simulink model "amplSim_2012b"  (R2012b)
settings: Solver=ode15s  StartTime=0.0  StopTime=30  RelTol=1e-6
values from neighbouring files (symbols this model uses):
  K = par(4)    [amplDiff.m]
  Qin = C*U    (= 2.912e-09)    [amplDiff.m]
  t0 = par(1)    [amplDiff.m]
  tau1 = par(2)    [amplDiff.m]
  tau2 = par(3)    [amplDiff.m]
  y_off = par(5)    [amplDiff.m]    (also in approxVol.m = theta(5))
settings Model: Creator=larer  LastModifiedBy=larer
settings DataIOCC: SignalLoggingSaveFormat=ModelDataLogs  SignalLoggingName=sigsOut
settings OptimizationCC: BooleanDataType=off  ExpressionDepthLimit=128
settings DebuggingCC: SaveWithParameterizedLinksMsg=none  SignalResolutionControl=TryResolveAllWithWarning  SolverPrmCheckMsg=none  MultiTaskDSMMsg=warning  MultiTaskCondExecSysMsg=none  FrameProcessingCompatibilityMsg=error  StateNameClashWarn=none  StrictBusMsg=None
settings HardwareCC: TargetUnknown=on
settings CodeAppCC: CustomSymbolStrType=$N$R$M_T
settings GRTTargetCC: CodeReplacementLibrary=C89/C90 (ANSI)  GeneratePreprocessorConditionals=Use local settings  CombineOutputUpdateFcns=off  GRTInterface=on

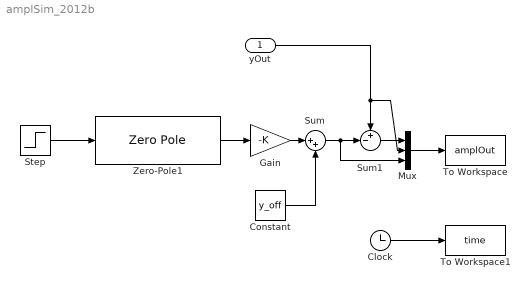
== system amplSim_2012b ==
  yOut : Inport
  Clock : Clock
  Constant : Constant  Value=y_off
  Gain : Gain  Gain=-K  SaturateOnIntegerOverflow=on  OutDataTypeStr=Inherit: Same as input  ParamDataTypeStr=Inherit: Same as input
  Mux : Mux  Inputs=3
  Step : Step  Time=t0  After=Qin  SampleTime=0
  Sum : Sum  Inputs=|++  SaturateOnIntegerOverflow=on  InputSameDT=on  OutDataTypeStr=Inherit: Same as first input
  Sum1 : Sum  Inputs=+-|  SaturateOnIntegerOverflow=on  InputSameDT=on  OutDataTypeStr=Inherit: Same as first input
  To Workspace : ToWorkspace  VariableName=amplOut  SampleTime=0.01
  To Workspace1 : ToWorkspace  VariableName=time  SampleTime=0.01
  Zero-Pole1 : ZeroPole  Zeros=[0]  Poles=[-1/tau1 -1/tau2]  Gain=[1/tau2/tau1]
  wires:
  Constant/1 -> Sum/2
  Gain/1 -> Sum/1
  Sum/1 -> Sum1/2, Mux/3
  yOut/1 -> Sum1/1, Mux/2
  Sum1/1 -> Mux/1
  Mux/1 -> To Workspace/1
  Clock/1 -> To Workspace1/1
  Step/1 -> Zero-Pole1/1
  Zero-Pole1/1 -> Gain/1
